simulink model "Project_template"  (R2014b)
settings: Solver=ode23tb  StartTime=0.0  StopTime=600  RelTol=1e-6  AbsTol=1e-6
values from neighbouring files (symbols this model uses):
  k = 1    [testfile.m]
  K_I = 0.03    [engine_sim.m]
  K_p = 0.002    [engine_sim.m]
undefined symbols (not defined in the file or in its folder): a_0, a_1, a_2, AFs, AirStep, alpha_REF_manual, alphaEND, alphaINI, alphaST, Boost_control, C_2, C_d, c_fi, c_fr_0, c_r1, c_r2, dp_thrREF, gamma_air, KiDriver, KpDriver, KpThr, KpWg, n_0, n_1, n_2, n_cyl, N_e_manual, N_e_step, n_ig_ch, n_r, NEND, NeST, Newton, NINI, p_amb, pedEND, pedINI, pedPos_manual, pedST, q_LHV, R_air, r_c, R_exh, Raphson, rho_air, rTurb, t_0, T_0, T_amb, T_hat_bef_thr, T_hat_im, T_ic, T_t, tau_d_bc, tau_th, TiThr, TiWg, V_d, V_D, V_em ... (+10)
libraries: simulink x1
(part 2 of 2)

== system Project_template/Engine/Turbocharger/Turbine/Tt ==
  Tem [K] : Inport
  etaT : Inport  Port=2
  PiT : Inport  Port=3
  Ground1 : Ground
  Terminator1 : Terminator
  Terminator2 : Terminator
  Terminator3 : Terminator
  Tt [K] : Outport
  wires:
  PiT/1 -> Terminator3/1
  etaT/1 -> Terminator2/1
  Tem [K]/1 -> Terminator1/1
  Ground1/1 -> Tt [K]/1

== system Project_template/Engine/Turbocharger/Turbine/etaT ==
  BSR : Inport
  Ground1 : Ground
  Max : MinMax  Function=max  Inputs=2
  Terminator1 : Terminator
  etaTmin : Constant  Value=0.3
  etaT : Outport
  wires:
  Max/1 -> etaT/1
  etaTmin/1 -> Max/2
  BSR/1 -> Terminator1/1
  Ground1/1 -> Max/1
